simulink model "twinconverter_lglfault_nonlinearload"  (Simulink 7.5)
settings: Solver=ode23tb  StartTime=0.0  StopTime=0.5  MaxStep=1e-5  RelTol=1e-4
libraries: powerlib x36, powerlib_extras x3, powerlib_models x1
(part 2 of 2)

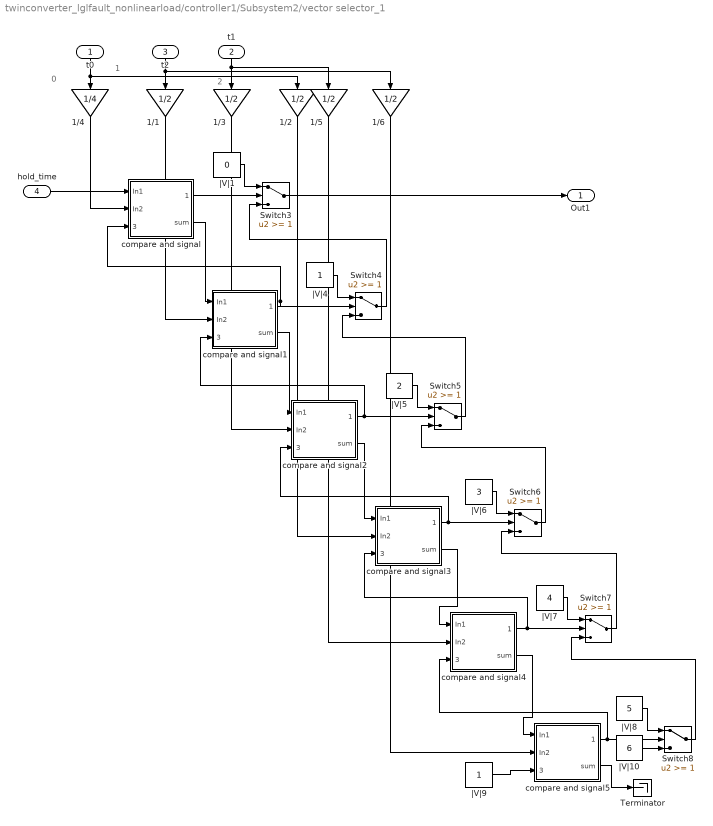
== system twinconverter_lglfault_nonlinearload/controller1/Subsystem2/vector selector_1 ==
  note: 0
  note: 1
  note: 2
  t0 : Inport
  t1 : Inport  Port=2
  t2 : Inport  Port=3
  hold_time : Inport  Port=4
  1/{1..3,5..6} (5 alike) : Gain  Gain=1/2  ParameterDataType=sfix(16)  ParameterScaling=2^0  OutDataType=sfix(16)  OutScaling=2^0
  1/4 : Gain  Gain=1/4  ParameterDataType=sfix(16)  ParameterScaling=2^0  OutDataType=sfix(16)  OutScaling=2^0
  Switch{3..8} (6 alike) : Switch  Threshold=1
  Terminator : Terminator
  compare and signal : Subsystem
  compare and signal1 : Subsystem
  compare and signal2 : Subsystem
  compare and signal3 : Subsystem
  compare and signal4 : Subsystem
  compare and signal5 : Subsystem
  |V|1 : Constant  Value=0  OutDataType=sfix(16)  OutScaling=2^0
  |V|10 : Constant  Value=6  OutDataType=sfix(16)  OutScaling=2^0
  |V|4 : Constant  OutDataType=sfix(16)  OutScaling=2^0
  |V|5 : Constant  Value=2  OutDataType=sfix(16)  OutScaling=2^0
  |V|6 : Constant  Value=3  OutDataType=sfix(16)  OutScaling=2^0
  |V|7 : Constant  Value=4  OutDataType=sfix(16)  OutScaling=2^0
  |V|8 : Constant  Value=5  OutDataType=sfix(16)  OutScaling=2^0
  |V|9 : Constant  OutDataType=sfix(16)  OutScaling=2^0
  Out1 : Outport
  wires:
  1/4/1 -> compare and signal/2(In2)
  t2/1 -> 1/1/1, 1/6/1
  t1/1 -> 1/3/1, 1/5/1
  t0/1 -> 1/4/1, 1/2/1
  hold_time/1 -> compare and signal/1(In1)
  compare and signal/1(logic_out) -> Switch3/2
  |V|1/1 -> Switch3/1
  compare and signal1/1(logic_out) -> compare and signal/3(logic_in), Switch4/2
  compare and signal/2(sum) -> compare and signal1/1(In1)
  1/1/1 -> compare and signal1/2(In2)
  |V|4/1 -> Switch4/1
  compare and signal1/2(sum) -> compare and signal2/1(In1)
  1/3/1 -> compare and signal2/2(In2)
  |V|5/1 -> Switch5/1
  compare and signal2/1(logic_out) -> Switch5/2, compare and signal1/3(logic_in)
  compare and signal2/2(sum) -> compare and signal3/1(In1)
  1/2/1 -> compare and signal3/2(In2)
  |V|6/1 -> Switch6/1
  compare and signal3/1(logic_out) -> Switch6/2, compare and signal2/3(logic_in)
  compare and signal3/2(sum) -> compare and signal4/1(In1)
  1/5/1 -> compare and signal4/2(In2)
  |V|7/1 -> Switch7/1
  compare and signal4/1(logic_out) -> Switch7/2, compare and signal3/3(logic_in)
  1/6/1 -> compare and signal5/2(In2)
  compare and signal4/2(sum) -> compare and signal5/1(In1)
  |V|8/1 -> Switch8/1
  compare and signal5/1(logic_out) -> Switch8/2, compare and signal4/3(logic_in)
  |V|9/1 -> compare and signal5/3(logic_in)
  |V|10/1 -> Switch8/3
  compare and signal5/2(sum) -> Terminator/1
  Switch8/1 -> Switch7/3
  Switch7/1 -> Switch6/3
  Switch6/1 -> Switch5/3
  Switch5/1 -> Switch4/3
  Switch4/1 -> Switch3/3
  Switch3/1 -> Out1/1

== system twinconverter_lglfault_nonlinearload/controller1/Subsystem1/vector selector_0/compare and signal ==
  In1 : Inport
  In2 : Inport  Port=2
  logic_in : Inport  Port=3
  " 2" : Logic  AllPortsSameDT=off  OutDataTypeMode=boolean  OutDataTypeStr=boolean
  Clock1 : Clock
      settings: Decimation=10
  Relational Operator3 : RelationalOperator  LogicOutDataTypeMode=boolean  OutDataTypeStr=boolean
  Sum1 : Sum  Inputs=++|  OutDataType=sfix(16)  OutScaling=2^0
  logic_out : Outport
  sum : Outport  Port=2
  wires:
  Sum1/1 -> Relational Operator3/1, sum/1
  Clock1/1 -> Relational Operator3/2
  Relational Operator3/1 -> " 2"/1
  In1/1 -> Sum1/1
  In2/1 -> Sum1/2
  " 2"/1 -> logic_out/1
  logic_in/1 -> " 2"/2

== system twinconverter_lglfault_nonlinearload/controller1/Subsystem1/vector selector_0/compare and signal1 ==
  In1 : Inport
  In2 : Inport  Port=2
  logic_in : Inport  Port=3
  " 2" : Logic  AllPortsSameDT=off  OutDataTypeMode=boolean  OutDataTypeStr=boolean
  Clock1 : Clock
      settings: Decimation=10
  Relational Operator3 : RelationalOperator  LogicOutDataTypeMode=boolean  OutDataTypeStr=boolean
  Sum1 : Sum  Inputs=++|  OutDataType=sfix(16)  OutScaling=2^0
  logic_out : Outport
  sum : Outport  Port=2
  wires:
  logic_in/1 -> " 2"/2
  " 2"/1 -> logic_out/1
  In2/1 -> Sum1/2
  In1/1 -> Sum1/1
  Relational Operator3/1 -> " 2"/1
  Clock1/1 -> Relational Operator3/2
  Sum1/1 -> sum/1, Relational Operator3/1

== system twinconverter_lglfault_nonlinearload/controller1/Subsystem1/vector selector_0/compare and signal2 ==
  In1 : Inport
  In2 : Inport  Port=2
  logic_in : Inport  Port=3
  " 2" : Logic  AllPortsSameDT=off  OutDataTypeMode=boolean  OutDataTypeStr=boolean
  Clock1 : Clock
      settings: Decimation=10
  Relational Operator3 : RelationalOperator  LogicOutDataTypeMode=boolean  OutDataTypeStr=boolean
  Sum1 : Sum  Inputs=++|  OutDataType=sfix(16)  OutScaling=2^0
  logic_out : Outport
  sum : Outport  Port=2
  wires:
  Sum1/1 -> Relational Operator3/1, sum/1
  Clock1/1 -> Relational Operator3/2
  Relational Operator3/1 -> " 2"/1
  In1/1 -> Sum1/1
  In2/1 -> Sum1/2
  " 2"/1 -> logic_out/1
  logic_in/1 -> " 2"/2

== system twinconverter_lglfault_nonlinearload/controller1/Subsystem1/vector selector_0/compare and signal3 ==
  In1 : Inport
  In2 : Inport  Port=2
  logic_in : Inport  Port=3
  " 2" : Logic  AllPortsSameDT=off  OutDataTypeMode=boolean  OutDataTypeStr=boolean
  Clock1 : Clock
      settings: Decimation=10
  Relational Operator3 : RelationalOperator  LogicOutDataTypeMode=boolean  OutDataTypeStr=boolean
  Sum1 : Sum  Inputs=++|  OutDataType=sfix(16)  OutScaling=2^0
  logic_out : Outport
  sum : Outport  Port=2
  wires:
  logic_in/1 -> " 2"/2
  " 2"/1 -> logic_out/1
  In2/1 -> Sum1/2
  In1/1 -> Sum1/1
  Relational Operator3/1 -> " 2"/1
  Clock1/1 -> Relational Operator3/2
  Sum1/1 -> sum/1, Relational Operator3/1

== system twinconverter_lglfault_nonlinearload/controller1/Subsystem1/vector selector_0/compare and signal4 ==
  In1 : Inport
  In2 : Inport  Port=2
  logic_in : Inport  Port=3
  " 2" : Logic  AllPortsSameDT=off  OutDataTypeMode=boolean  OutDataTypeStr=boolean
  Clock1 : Clock
      settings: Decimation=10
  Relational Operator3 : RelationalOperator  LogicOutDataTypeMode=boolean  OutDataTypeStr=boolean
  Sum1 : Sum  Inputs=++|  OutDataType=sfix(16)  OutScaling=2^0
  logic_out : Outport
  sum : Outport  Port=2
  wires:
  Sum1/1 -> Relational Operator3/1, sum/1
  Clock1/1 -> Relational Operator3/2
  Relational Operator3/1 -> " 2"/1
  In1/1 -> Sum1/1
  In2/1 -> Sum1/2
  " 2"/1 -> logic_out/1
  logic_in/1 -> " 2"/2

== system twinconverter_lglfault_nonlinearload/controller1/Subsystem1/vector selector_0/compare and signal5 ==
  In1 : Inport
  In2 : Inport  Port=2
  logic_in : Inport  Port=3
  " 2" : Logic  AllPortsSameDT=off  OutDataTypeMode=boolean  OutDataTypeStr=boolean
  Clock1 : Clock
      settings: Decimation=10
  Relational Operator3 : RelationalOperator  LogicOutDataTypeMode=boolean  OutDataTypeStr=boolean
  Sum1 : Sum  Inputs=++|  OutDataType=sfix(16)  OutScaling=2^0
  logic_out : Outport
  sum : Outport  Port=2
  wires:
  Sum1/1 -> Relational Operator3/1, sum/1
  Clock1/1 -> Relational Operator3/2
  Relational Operator3/1 -> " 2"/1
  In1/1 -> Sum1/1
  In2/1 -> Sum1/2
  " 2"/1 -> logic_out/1
  logic_in/1 -> " 2"/2

== system twinconverter_lglfault_nonlinearload/controller1/Subsystem1/vector selector_1/compare and signal ==
  In1 : Inport
  In2 : Inport  Port=2
  logic_in : Inport  Port=3
  " 2" : Logic  AllPortsSameDT=off  OutDataTypeMode=boolean  OutDataTypeStr=boolean
  Clock1 : Clock
      settings: Decimation=10
  Relational Operator3 : RelationalOperator  LogicOutDataTypeMode=boolean  OutDataTypeStr=boolean
  Sum1 : Sum  Inputs=++|  OutDataType=sfix(16)  OutScaling=2^0
  logic_out : Outport
  sum : Outport  Port=2
  wires:
  logic_in/1 -> " 2"/2
  " 2"/1 -> logic_out/1
  In2/1 -> Sum1/2
  In1/1 -> Sum1/1
  Relational Operator3/1 -> " 2"/1
  Clock1/1 -> Relational Operator3/2
  Sum1/1 -> sum/1, Relational Operator3/1

== system twinconverter_lglfault_nonlinearload/controller1/Subsystem1/vector selector_1/compare and signal1 ==
  In1 : Inport
  In2 : Inport  Port=2
  logic_in : Inport  Port=3
  " 2" : Logic  AllPortsSameDT=off  OutDataTypeMode=boolean  OutDataTypeStr=boolean
  Clock1 : Clock
      settings: Decimation=10
  Relational Operator3 : RelationalOperator  LogicOutDataTypeMode=boolean  OutDataTypeStr=boolean
  Sum1 : Sum  Inputs=++|  OutDataType=sfix(16)  OutScaling=2^0
  logic_out : Outport
  sum : Outport  Port=2
  wires:
  Sum1/1 -> Relational Operator3/1, sum/1
  Clock1/1 -> Relational Operator3/2
  Relational Operator3/1 -> " 2"/1
  In1/1 -> Sum1/1
  In2/1 -> Sum1/2
  " 2"/1 -> logic_out/1
  logic_in/1 -> " 2"/2

== system twinconverter_lglfault_nonlinearload/controller1/Subsystem1/vector selector_1/compare and signal2 ==
  In1 : Inport
  In2 : Inport  Port=2
  logic_in : Inport  Port=3
  " 2" : Logic  AllPortsSameDT=off  OutDataTypeMode=boolean  OutDataTypeStr=boolean
  Clock1 : Clock
      settings: Decimation=10
  Relational Operator3 : RelationalOperator  LogicOutDataTypeMode=boolean  OutDataTypeStr=boolean
  Sum1 : Sum  Inputs=++|  OutDataType=sfix(16)  OutScaling=2^0
  logic_out : Outport
  sum : Outport  Port=2
  wires:
  logic_in/1 -> " 2"/2
  " 2"/1 -> logic_out/1
  In2/1 -> Sum1/2
  In1/1 -> Sum1/1
  Relational Operator3/1 -> " 2"/1
  Clock1/1 -> Relational Operator3/2
  Sum1/1 -> sum/1, Relational Operator3/1

== system twinconverter_lglfault_nonlinearload/controller1/Subsystem1/vector selector_1/compare and signal3 ==
  In1 : Inport
  In2 : Inport  Port=2
  logic_in : Inport  Port=3
  " 2" : Logic  AllPortsSameDT=off  OutDataTypeMode=boolean  OutDataTypeStr=boolean
  Clock1 : Clock
      settings: Decimation=10
  Relational Operator3 : RelationalOperator  LogicOutDataTypeMode=boolean  OutDataTypeStr=boolean
  Sum1 : Sum  Inputs=++|  OutDataType=sfix(16)  OutScaling=2^0
  logic_out : Outport
  sum : Outport  Port=2
  wires:
  Sum1/1 -> Relational Operator3/1, sum/1
  Clock1/1 -> Relational Operator3/2
  Relational Operator3/1 -> " 2"/1
  In1/1 -> Sum1/1
  In2/1 -> Sum1/2
  " 2"/1 -> logic_out/1
  logic_in/1 -> " 2"/2

== system twinconverter_lglfault_nonlinearload/controller1/Subsystem1/vector selector_1/compare and signal4 ==
  In1 : Inport
  In2 : Inport  Port=2
  logic_in : Inport  Port=3
  " 2" : Logic  AllPortsSameDT=off  OutDataTypeMode=boolean  OutDataTypeStr=boolean
  Clock1 : Clock
      settings: Decimation=10
  Relational Operator3 : RelationalOperator  LogicOutDataTypeMode=boolean  OutDataTypeStr=boolean
  Sum1 : Sum  Inputs=++|  OutDataType=sfix(16)  OutScaling=2^0
  logic_out : Outport
  sum : Outport  Port=2
  wires:
  logic_in/1 -> " 2"/2
  " 2"/1 -> logic_out/1
  In2/1 -> Sum1/2
  In1/1 -> Sum1/1
  Relational Operator3/1 -> " 2"/1
  Clock1/1 -> Relational Operator3/2
  Sum1/1 -> sum/1, Relational Operator3/1

== system twinconverter_lglfault_nonlinearload/controller1/Subsystem1/vector selector_1/compare and signal5 ==
  In1 : Inport
  In2 : Inport  Port=2
  logic_in : Inport  Port=3
  " 2" : Logic  AllPortsSameDT=off  OutDataTypeMode=boolean  OutDataTypeStr=boolean
  Clock1 : Clock
      settings: Decimation=10
  Relational Operator3 : RelationalOperator  LogicOutDataTypeMode=boolean  OutDataTypeStr=boolean
  Sum1 : Sum  Inputs=++|  OutDataType=sfix(16)  OutScaling=2^0
  logic_out : Outport
  sum : Outport  Port=2
  wires:
  logic_in/1 -> " 2"/2
  " 2"/1 -> logic_out/1
  In2/1 -> Sum1/2
  In1/1 -> Sum1/1
  Relational Operator3/1 -> " 2"/1
  Clock1/1 -> Relational Operator3/2
  Sum1/1 -> sum/1, Relational Operator3/1

== system twinconverter_lglfault_nonlinearload/controller1/Subsystem2/vector selector_0/compare and signal ==
  In1 : Inport
  In2 : Inport  Port=2
  logic_in : Inport  Port=3
  " 2" : Logic  AllPortsSameDT=off  OutDataTypeMode=boolean  OutDataTypeStr=boolean
  Clock1 : Clock
      settings: Decimation=10
  Relational Operator3 : RelationalOperator  LogicOutDataTypeMode=boolean  OutDataTypeStr=boolean
  Sum1 : Sum  Inputs=++|  OutDataType=sfix(16)  OutScaling=2^0
  logic_out : Outport
  sum : Outport  Port=2
  wires:
  logic_in/1 -> " 2"/2
  " 2"/1 -> logic_out/1
  In2/1 -> Sum1/2
  In1/1 -> Sum1/1
  Relational Operator3/1 -> " 2"/1
  Clock1/1 -> Relational Operator3/2
  Sum1/1 -> sum/1, Relational Operator3/1

== system twinconverter_lglfault_nonlinearload/controller1/Subsystem2/vector selector_0/compare and signal1 ==
  In1 : Inport
  In2 : Inport  Port=2
  logic_in : Inport  Port=3
  " 2" : Logic  AllPortsSameDT=off  OutDataTypeMode=boolean  OutDataTypeStr=boolean
  Clock1 : Clock
      settings: Decimation=10
  Relational Operator3 : RelationalOperator  LogicOutDataTypeMode=boolean  OutDataTypeStr=boolean
  Sum1 : Sum  Inputs=++|  OutDataType=sfix(16)  OutScaling=2^0
  logic_out : Outport
  sum : Outport  Port=2
  wires:
  Sum1/1 -> Relational Operator3/1, sum/1
  Clock1/1 -> Relational Operator3/2
  Relational Operator3/1 -> " 2"/1
  In1/1 -> Sum1/1
  In2/1 -> Sum1/2
  " 2"/1 -> logic_out/1
  logic_in/1 -> " 2"/2

== system twinconverter_lglfault_nonlinearload/controller1/Subsystem2/vector selector_0/compare and signal2 ==
  In1 : Inport
  In2 : Inport  Port=2
  logic_in : Inport  Port=3
  " 2" : Logic  AllPortsSameDT=off  OutDataTypeMode=boolean  OutDataTypeStr=boolean
  Clock1 : Clock
      settings: Decimation=10
  Relational Operator3 : RelationalOperator  LogicOutDataTypeMode=boolean  OutDataTypeStr=boolean
  Sum1 : Sum  Inputs=++|  OutDataType=sfix(16)  OutScaling=2^0
  logic_out : Outport
  sum : Outport  Port=2
  wires:
  logic_in/1 -> " 2"/2
  " 2"/1 -> logic_out/1
  In2/1 -> Sum1/2
  In1/1 -> Sum1/1
  Relational Operator3/1 -> " 2"/1
  Clock1/1 -> Relational Operator3/2
  Sum1/1 -> sum/1, Relational Operator3/1

== system twinconverter_lglfault_nonlinearload/controller1/Subsystem2/vector selector_0/compare and signal3 ==
  In1 : Inport
  In2 : Inport  Port=2
  logic_in : Inport  Port=3
  " 2" : Logic  AllPortsSameDT=off  OutDataTypeMode=boolean  OutDataTypeStr=boolean
  Clock1 : Clock
      settings: Decimation=10
  Relational Operator3 : RelationalOperator  LogicOutDataTypeMode=boolean  OutDataTypeStr=boolean
  Sum1 : Sum  Inputs=++|  OutDataType=sfix(16)  OutScaling=2^0
  logic_out : Outport
  sum : Outport  Port=2
  wires:
  Sum1/1 -> Relational Operator3/1, sum/1
  Clock1/1 -> Relational Operator3/2
  Relational Operator3/1 -> " 2"/1
  In1/1 -> Sum1/1
  In2/1 -> Sum1/2
  " 2"/1 -> logic_out/1
  logic_in/1 -> " 2"/2

== system twinconverter_lglfault_nonlinearload/controller1/Subsystem2/vector selector_0/compare and signal4 ==
  In1 : Inport
  In2 : Inport  Port=2
  logic_in : Inport  Port=3
  " 2" : Logic  AllPortsSameDT=off  OutDataTypeMode=boolean  OutDataTypeStr=boolean
  Clock1 : Clock
      settings: Decimation=10
  Relational Operator3 : RelationalOperator  LogicOutDataTypeMode=boolean  OutDataTypeStr=boolean
  Sum1 : Sum  Inputs=++|  OutDataType=sfix(16)  OutScaling=2^0
  logic_out : Outport
  sum : Outport  Port=2
  wires:
  logic_in/1 -> " 2"/2
  " 2"/1 -> logic_out/1
  In2/1 -> Sum1/2
  In1/1 -> Sum1/1
  Relational Operator3/1 -> " 2"/1
  Clock1/1 -> Relational Operator3/2
  Sum1/1 -> sum/1, Relational Operator3/1

== system twinconverter_lglfault_nonlinearload/controller1/Subsystem2/vector selector_0/compare and signal5 ==
  In1 : Inport
  In2 : Inport  Port=2
  logic_in : Inport  Port=3
  " 2" : Logic  AllPortsSameDT=off  OutDataTypeMode=boolean  OutDataTypeStr=boolean
  Clock1 : Clock
      settings: Decimation=10
  Relational Operator3 : RelationalOperator  LogicOutDataTypeMode=boolean  OutDataTypeStr=boolean
  Sum1 : Sum  Inputs=++|  OutDataType=sfix(16)  OutScaling=2^0
  logic_out : Outport
  sum : Outport  Port=2
  wires:
  logic_in/1 -> " 2"/2
  " 2"/1 -> logic_out/1
  In2/1 -> Sum1/2
  In1/1 -> Sum1/1
  Relational Operator3/1 -> " 2"/1
  Clock1/1 -> Relational Operator3/2
  Sum1/1 -> sum/1, Relational Operator3/1

== system twinconverter_lglfault_nonlinearload/controller1/Subsystem2/vector selector_1/compare and signal ==
  In1 : Inport
  In2 : Inport  Port=2
  logic_in : Inport  Port=3
  " 2" : Logic  AllPortsSameDT=off  OutDataTypeMode=boolean  OutDataTypeStr=boolean
  Clock1 : Clock
      settings: Decimation=10
  Relational Operator3 : RelationalOperator  LogicOutDataTypeMode=boolean  OutDataTypeStr=boolean
  Sum1 : Sum  Inputs=++|  OutDataType=sfix(16)  OutScaling=2^0
  logic_out : Outport
  sum : Outport  Port=2
  wires:
  Sum1/1 -> Relational Operator3/1, sum/1
  Clock1/1 -> Relational Operator3/2
  Relational Operator3/1 -> " 2"/1
  In1/1 -> Sum1/1
  In2/1 -> Sum1/2
  " 2"/1 -> logic_out/1
  logic_in/1 -> " 2"/2

== system twinconverter_lglfault_nonlinearload/controller1/Subsystem2/vector selector_1/compare and signal1 ==
  In1 : Inport
  In2 : Inport  Port=2
  logic_in : Inport  Port=3
  " 2" : Logic  AllPortsSameDT=off  OutDataTypeMode=boolean  OutDataTypeStr=boolean
  Clock1 : Clock
      settings: Decimation=10
  Relational Operator3 : RelationalOperator  LogicOutDataTypeMode=boolean  OutDataTypeStr=boolean
  Sum1 : Sum  Inputs=++|  OutDataType=sfix(16)  OutScaling=2^0
  logic_out : Outport
  sum : Outport  Port=2
  wires:
  logic_in/1 -> " 2"/2
  " 2"/1 -> logic_out/1
  In2/1 -> Sum1/2
  In1/1 -> Sum1/1
  Relational Operator3/1 -> " 2"/1
  Clock1/1 -> Relational Operator3/2
  Sum1/1 -> sum/1, Relational Operator3/1

== system twinconverter_lglfault_nonlinearload/controller1/Subsystem2/vector selector_1/compare and signal2 ==
  In1 : Inport
  In2 : Inport  Port=2
  logic_in : Inport  Port=3
  " 2" : Logic  AllPortsSameDT=off  OutDataTypeMode=boolean  OutDataTypeStr=boolean
  Clock1 : Clock
      settings: Decimation=10
  Relational Operator3 : RelationalOperator  LogicOutDataTypeMode=boolean  OutDataTypeStr=boolean
  Sum1 : Sum  Inputs=++|  OutDataType=sfix(16)  OutScaling=2^0
  logic_out : Outport
  sum : Outport  Port=2
  wires:
  Sum1/1 -> Relational Operator3/1, sum/1
  Clock1/1 -> Relational Operator3/2
  Relational Operator3/1 -> " 2"/1
  In1/1 -> Sum1/1
  In2/1 -> Sum1/2
  " 2"/1 -> logic_out/1
  logic_in/1 -> " 2"/2

== system twinconverter_lglfault_nonlinearload/controller1/Subsystem2/vector selector_1/compare and signal3 ==
  In1 : Inport
  In2 : Inport  Port=2
  logic_in : Inport  Port=3
  " 2" : Logic  AllPortsSameDT=off  OutDataTypeMode=boolean  OutDataTypeStr=boolean
  Clock1 : Clock
      settings: Decimation=10
  Relational Operator3 : RelationalOperator  LogicOutDataTypeMode=boolean  OutDataTypeStr=boolean
  Sum1 : Sum  Inputs=++|  OutDataType=sfix(16)  OutScaling=2^0
  logic_out : Outport
  sum : Outport  Port=2
  wires:
  logic_in/1 -> " 2"/2
  " 2"/1 -> logic_out/1
  In2/1 -> Sum1/2
  In1/1 -> Sum1/1
  Relational Operator3/1 -> " 2"/1
  Clock1/1 -> Relational Operator3/2
  Sum1/1 -> sum/1, Relational Operator3/1

== system twinconverter_lglfault_nonlinearload/controller1/Subsystem2/vector selector_1/compare and signal4 ==
  In1 : Inport
  In2 : Inport  Port=2
  logic_in : Inport  Port=3
  " 2" : Logic  AllPortsSameDT=off  OutDataTypeMode=boolean  OutDataTypeStr=boolean
  Clock1 : Clock
      settings: Decimation=10
  Relational Operator3 : RelationalOperator  LogicOutDataTypeMode=boolean  OutDataTypeStr=boolean
  Sum1 : Sum  Inputs=++|  OutDataType=sfix(16)  OutScaling=2^0
  logic_out : Outport
  sum : Outport  Port=2
  wires:
  Sum1/1 -> Relational Operator3/1, sum/1
  Clock1/1 -> Relational Operator3/2
  Relational Operator3/1 -> " 2"/1
  In1/1 -> Sum1/1
  In2/1 -> Sum1/2
  " 2"/1 -> logic_out/1
  logic_in/1 -> " 2"/2

== system twinconverter_lglfault_nonlinearload/controller1/Subsystem2/vector selector_1/compare and signal5 ==
  In1 : Inport
  In2 : Inport  Port=2
  logic_in : Inport  Port=3
  " 2" : Logic  AllPortsSameDT=off  OutDataTypeMode=boolean  OutDataTypeStr=boolean
  Clock1 : Clock
      settings: Decimation=10
  Relational Operator3 : RelationalOperator  LogicOutDataTypeMode=boolean  OutDataTypeStr=boolean
  Sum1 : Sum  Inputs=++|  OutDataType=sfix(16)  OutScaling=2^0
  logic_out : Outport
  sum : Outport  Port=2
  wires:
  Sum1/1 -> Relational Operator3/1, sum/1
  Clock1/1 -> Relational Operator3/2
  Relational Operator3/1 -> " 2"/1
  In1/1 -> Sum1/1
  In2/1 -> Sum1/2
  " 2"/1 -> logic_out/1
  logic_in/1 -> " 2"/2
